simulink model "test"  (R2020a)
settings: Solver=VariableStepAuto  StartTime=0.0  StopTime=1  RelTol=1e-3
model workspace (MAT data in the model file):
  X1 = 1.102
libraries: powerlib x4, simulink x2
settings Model: ParameterArgumentNames=X1  OrderedModelArguments=off  Creator=adam_  LastModifiedBy=j_temriv

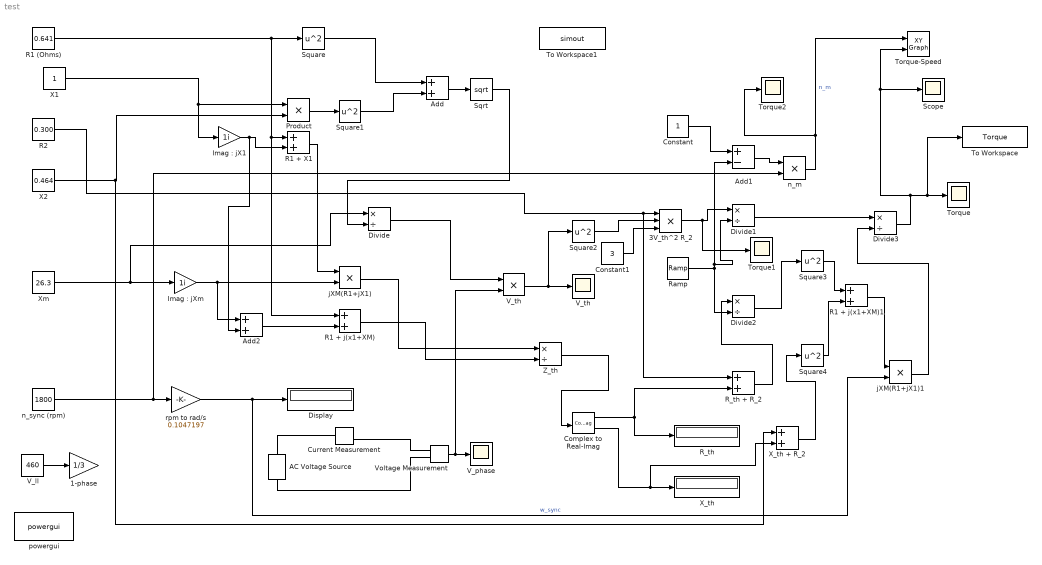
== system test ==
  1-phase : Gain  Gain=1/3
  3V_th^2 R_2 : Product  Inputs=3
  AC Voltage Source : powerlib/Electrical Sources/AC Voltage Source  Amplitude=153.33  Phase=0  Frequency=60  SampleTime=0.0001  Measurements=None  BusType=swing  Pref=10e3  Qref=0  Qmin=-inf  Qmax=+inf
  Add : Sum
  Add1 : Sum  Inputs=+-
  Add2 : Sum
  Complex to Real-Imag : ComplexToRealImag
  Constant : Constant
  Constant1 : Constant  Value=3
  Current Measurement : powerlib/Measurements/Current Measurement  PhasorSimulation=off  OutputType=Complex  PSBequivalent=0
  Display : Display
  Divide{,1..3} (4 alike) : Product  Inputs=*/
  "Imag : jX1" : Gain  Gain=1i
  "Imag : jXm" : Gain  Gain=1i
  Product : Product
  R1 (Ohms) : Constant  Value=0.641
  R1 + X1 : Sum
  R1 + j(x1+XM) : Sum
  R1 + j(x1+XM)1 : Sum
  "R2 " : Constant  Value=0.300
  R_th : Display
  R_th + R_2 : Sum
  Ramp : simulink/Sources/Ramp  slope=1  start=0  InitialOutput=0.001
  Scope : Scope
  Sqrt : Sqrt  SaturateOnIntegerOverflow=on
  Square{,1..4} (5 alike) : Math  Operator=square  SaturateOnIntegerOverflow=on
  To Workspace : ToWorkspace  VariableName=Torque  SaveFormat=Timeseries  SampleTime=-1
  To Workspace1 : ToWorkspace  VariableName=simout  SaveFormat=Timeseries  SampleTime=-1
  Torque : Scope
  Torque-Speed : simulink/Sinks/XY Graph  xmin=0  xmax=1950  ymin=0  ymax=50000  st=-1
  Torque1 : Scope
  Torque2 : Scope
  V_ll : Constant  Value=460
  V_phase : Scope
  V_th : Scope
  "V_th " : Product
  Voltage Measurement : powerlib/Measurements/Voltage Measurement  PhasorSimulation=off  OutputType=Complex  PSBequivalent=0
  X1 : Constant
  X2 : Constant  Value=0.464
  X_th : Display
  X_th + R_2 : Sum
  "Xm " : Constant  Value=26.3
  Z_th : Product  Inputs=*/
  jXM(R1+jX1) : Product
  jXM(R1+jX1)1 : Product
  n_m : Product
  n_sync (rpm) : Constant  Value=1800
  powergui : powerlib/powergui  Priority=1  SimulationMode=Continuous  SampleTime=50e-6  frequency=60  Iterations=50  frequencyindice=60  Pbase=100e6  ErrMax=1e-4  UnitsV=kV  UnitsW=MW  buscounter=0  FunctionMessages=off  echomessages=off  EnableUseOfTLC=off  CurrentSourceSwitches=off  DisableSnubberDevices=off  DisableRonSwitches=off  DisableVfSwitches=off  DisplayEquations=off  AutomaticDiscreteSolvers=off  SolverType=Tustin/Backward Euler (TBE)  Interpol=off  ExternalGateDelay=off  methode=off  Ts=100  x0status=blocks  SPID=on  SwTol=0  HookPort=off  NonlinearTolerance=1e-4  nMaxIteration=100  ContinueOnMaxIteration=off  RestoreLinks=warning  ResistiveCurrentMeasurement=off  Frange=[0:2:500]  Ylog=off  Xlog=on  ShowGrid=off  save=off  variable=ZData  structure=0  ZoomFFT=off  StartTime=0.0  cycles=1  DisplayStyle=1  fundamental=60  FreqAxis=off  MaxFrequency=1000  frequencyindicesteady=1  RmsSteady=1  display=off
  rpm to rad/s : Gain  Gain=0.1047197
  wires:
  X2/1 -> X_th + R_2/1, Product/2
  R1 (Ohms)/1 -> R1 + j(x1+XM)/1, R1 + X1/1, Square/1
  "Xm "/1 -> "Imag : jXm"/1, Divide/1
  n_sync (rpm)/1 -> n_m/2, rpm to rad/s/1
  rpm to rad/s/1 -> jXM(R1+jX1)1/2, Display/1  "w_sync"
  Product/1 -> Square1/1
  Add/1 -> Sqrt/1
  Square/1 -> Add/1
  Square1/1 -> Add/2
  Sqrt/1 -> Divide/2
  Divide/1 -> "V_th "/1
  "Imag : jX1"/1 -> Add2/2, R1 + X1/2
  R1 + X1/1 -> jXM(R1+jX1)/1
  Z_th/1 -> Complex to Real-Imag/1
  "Imag : jXm"/1 -> Add2/1, jXM(R1+jX1)/2
  Add2/1 -> R1 + j(x1+XM)/2
  R1 + j(x1+XM)/1 -> Z_th/2
  jXM(R1+jX1)/1 -> Z_th/1
  Complex to Real-Imag/1 -> R_th/1, R_th + R_2/2
  Complex to Real-Imag/2 -> X_th + R_2/2, X_th/1
  "V_th "/1 -> V_th/1, Square2/1
  Square2/1 -> 3V_th^2 R_2/2
  "R2 "/1 -> R_th + R_2/1, 3V_th^2 R_2/1
  Ramp/1 -> Add1/2, Divide1/2, Divide2/2
  3V_th^2 R_2/1 -> Torque1/1, Divide1/1
  R_th + R_2/1 -> Divide2/1
  Divide2/1 -> Square3/1
  X_th + R_2/1 -> Square4/1
  Square3/1 -> R1 + j(x1+XM)1/1
  Square4/1 -> R1 + j(x1+XM)1/2
  R1 + j(x1+XM)1/1 -> jXM(R1+jX1)1/1
  jXM(R1+jX1)1/1 -> Divide3/2
  Divide1/1 -> Divide3/1
  Voltage Measurement/1 -> "V_th "/2, V_phase/1
  V_ll/1 -> 1-phase/1
  Divide3/1 -> To Workspace/1, Torque/1, Scope/1, Torque-Speed/2
  Constant/1 -> Add1/1
  Add1/1 -> n_m/1
  n_m/1 -> Torque2/1, Torque-Speed/1  "n_m"
  Constant1/1 -> 3V_th^2 R_2/3
  X1/1 -> "Imag : jX1"/1, Product/1
  connections:
  Current Measurement/RConn1 -- Voltage Measurement/LConn1
  Voltage Measurement/LConn2 -- AC Voltage Source/LConn1
  AC Voltage Source/RConn1 -- Current Measurement/LConn1
